simulink model "half_car_model_active_suspension_bump_brik"  (R2023b)
settings: Solver=VariableStepAuto  StartTime=0.0  StopTime=20  RelTol=1e-3
values from neighbouring files (symbols this model uses):
  e0 = [0; 0]    [half_car_active_suspensions_bump_brik.m]
  p = [ m ... (first row only)    [parameters.m]
  r0 = [Delta0 ... (first row only)    [half_car_active_suspensions_bump_brik.m]
  u0 = [0 ... (first row only)    [half_car_active_suspensions_bump_brik.m]    (also in prova_ordinata.m = [0; k * Delta0 * (df - dr)]; prova_ordinata_novembre.m = [0; k * Delta0 * (df - dr)])
  x0 = [Delta0 ... (first row only)    [half_car_active_suspensions_bump_brik.m]    (also in prova.m = [  -m*g/(2*k); prova_ordinata.m; prova_ordinata_novembre.m = [Delta0; 0; 0; 0; 0; 0; 0; 0])
  x0_lin = [ ... (first row only)    [half_car_active_suspensions_bump_brik.m]
  y0 = [0 ... (first row only)    [half_car_active_suspensions_bump_brik.m]
libraries: simulink x1
settings Model: Creator=alex2  LastModifiedBy=alex2

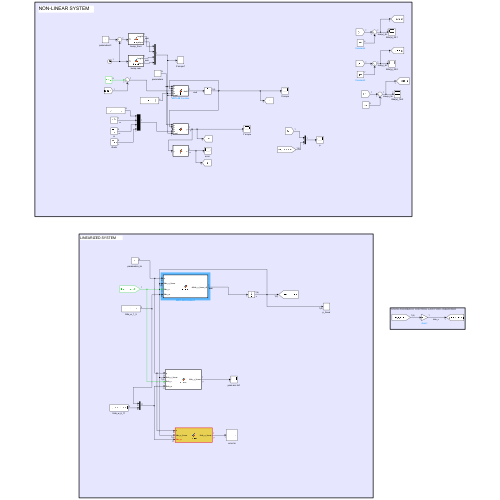
[thumbnail: Simulink's stored preview of the top-level diagram]
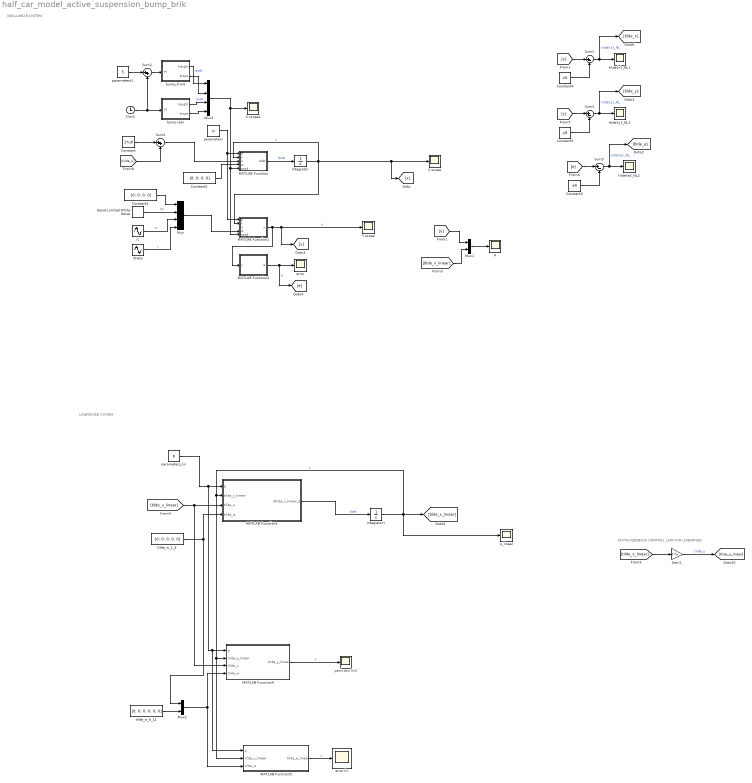
== system half_car_model_active_suspension_bump_brik ==
  note: LINEARIZED SYSTEM
  note: NON-LINEAR SYSTEM
  note: STATE-FEEDBACK CONTROL LAW FOR LINEARISED
  " error lin" : Scope
  Band-Limited White Noise : simulink/Sources/Band-Limited White Noise  Cov="1*[0.00001*1e-2; 0.00001*1e-2;  0.00001*1e-2; 0.00001*1e-2; 0.00001*1e-2]"  Ts=1e-2  seed=[23341; 31826; 11111; 81818; 00001]
  Clock : Clock
  Constant : Constant  Value=1*u0
  Constant1 : Constant  Value=[0; 0; 0; 0]
  Constant2 : Constant  Value=[0; 0; 0; 0]
  Constant3 : Constant  Value=y0
  Constant4 : Constant  Value=x0
  Constant5 : Constant  Value=e0
  Gain1 : Gain  Gain=0  Multiplication=Matrix(K*u)
  Integrator : Integrator  InitialCondition=x0
  Integrator1 : Integrator  InitialCondition=x0_lin
  MATLAB Function : MATLAB Function  TreatAsAtomicUnit=on
  MATLAB Function1 : MATLAB Function  TreatAsAtomicUnit=on
  MATLAB Function2 : MATLAB Function  TreatAsAtomicUnit=on
  MATLAB Function3 : MATLAB Function  TreatAsAtomicUnit=on
  MATLAB Function4 : MATLAB Function  TreatAsAtomicUnit=on
  MATLAB Function5 : MATLAB Function  TreatAsAtomicUnit=on
  Mux : Mux
  Mux1 : Mux  Inputs=2
  Mux2 : Mux  Inputs=2
  Mux3 : Mux
  Sum1 : Sum  Inputs=|+-
  Sum2 : Sum  Inputs=|++
  Sum3 : Sum  Inputs=|+-
  Sum4 : Sum  Inputs=|++
  Sum5 : Sum  Inputs=|+-
  X scope : Scope
  X scope1 : Scope
  Y scope : Scope
  bump rear : MATLAB Function  TreatAsAtomicUnit=on
  bump_front : MATLAB Function  TreatAsAtomicUnit=on
  "error " : Scope
  p : Scope
  p_linear : Scope
  parameters : Constant  Value=p
  parameters1 : Constant  Value=5
  parameters_lin : Constant  Value=p
  rtheta : Sin  Amplitude=0  Bias=r0  Frequency=0  SampleTime=0
  rz : Sin  Amplitude=0  Bias=r0  Frequency=0  SampleTime=0
  tilde_w_1_5 : Constant  Value=[0; 0; 0; 0; 0]
  tilde_w_6_11 : Constant  Value=[0; 0; 0; 0; 0; 0]
  "tilde{e}_NL2" : Scope
  "tilde{x}_NL1" : Scope
  "tilde{y}_NL2" : Scope
  yaxis acc lin1 : Scope
  wires:
  MATLAB Function/1(dxdt) -> Integrator/1  "dxdt"
  Integrator/1 -> MATLAB Function1/2(x), [x], X scope/1, MATLAB Function/2(x)  "x"
  Band-Limited White Noise/1 -> Mux/2  "nu"
  rz/1 -> Mux/3  "rz"
  Constant1/1 -> Mux/1
  Mux/1 -> MATLAB Function1/4(w)
  Constant2/1 -> MATLAB Function/4(w)
  MATLAB Function1/1(y) -> Y scope/1, [y], MATLAB Function2/1(y)  "y"
  rtheta/1 -> Mux/4  "r"
  MATLAB Function2/1(e) -> [e], "error "/1  "e"
  tilde_w_1_5/1 -> Mux2/1, MATLAB Function3/4(tilde_w)
  [tilde_u_linear] -> MATLAB Function4/3(tilde_u), MATLAB Function3/3(tilde_u)
  MATLAB Function3/1(dtilde_x_linear_dt) -> Integrator1/1  "dxdt"
  Integrator1/1 -> p_linear/1, MATLAB Function5/2(tilde_x_linear), MATLAB Function4/2(tilde_x_linear), MATLAB Function3/2(tilde_x_linear), [tilde_x_linear]  "x"
  parameters/1 -> MATLAB Function1/1(p), MATLAB Function/1(p)
  parameters_lin/1 -> MATLAB Function5/1(p), MATLAB Function4/1(p), MATLAB Function3/1(p)
  Mux2/1 -> MATLAB Function4/4(tilde_w), MATLAB Function5/3(tilde_w)
  tilde_w_6_11/1 -> Mux2/2
  MATLAB Function5/1(tilde_e_linear) -> " error lin"/1  "y"
  [tilde_u] -> Sum4/2
  Constant/1 -> Sum4/1
  Sum4/1 -> MATLAB Function/3(u)
  Sum1/1 -> [tilde_x], "tilde{x}_NL1"/1  "tilde{x}_NL"
  [x] -> Sum1/1
  Constant4/1 -> Sum1/2
  Gain1/1 -> [tilde_u_linear]  "tilde_u"
  [tilde_x_linear] -> Gain1/1
  MATLAB Function4/1(tilde_y_linear) -> yaxis acc lin1/1  "y"
  Mux1/1 -> p/1
  [x] -> Mux1/1
  [tilde_x_linear] -> Mux1/2
  Mux3/1 -> MATLAB Function/5(road), MATLAB Function1/5(road), X scope1/1
  Clock/1 -> Sum2/2, bump rear/1(Tf)
  bump rear/1(height) -> Mux3/3  "dxdt"
  bump rear/2(slope) -> Mux3/4
  bump_front/2(slope) -> Mux3/2
  bump_front/1(height) -> Mux3/1  "dxdt"
  Sum2/1 -> bump_front/1(Tf)
  parameters1/1 -> Sum2/1
  [y] -> Sum3/1
  Sum3/1 -> [tilde_y], "tilde{y}_NL2"/1  "tilde{y}_NL"
  Constant3/1 -> Sum3/2
  [e] -> Sum5/1
  Sum5/1 -> [tilde_e], "tilde{e}_NL2"/1  "tilde{e}_NL"
  Constant5/1 -> Sum5/2

== matlab function half_car_model_active_suspension_bump_brik/MATLAB Function1 ==
  data: p input; x input; u input; y output; w input; road input
function y = h(p,x, u, w, road)

%% parameters
m = p(1);      % [kg] mass
k = p(2);    % [N/m] spring stiffness
beta = p(3);   % [N/(m/s)] damper coeff.
ell0 = p(4);   % [m] 0-load lenght
g = p(5);   % [m/s^2] gravity acceleration
df = p(6);     % [m] distance between center of mass and front
dr = p(7);     % [m] distance between center of mass and rear
J = p(8);      % [kg*m^2] Moment of intertia

%% state
pz = x(1);        % [m] heigth of the center of mass of the car 
vz = x(2);        % [m/s] speed of the center of mass of the car 
ptheta = x(3);    % [Rad] pitch angle of the car 
vtheta = x(4);    % [Rad/s] angular speed of the car 
thetaroad_f = road(3); % [Rad]Road slope
zroad_f = road(4);     %[m]Road height 
thetaroad_r = -road(1); % [Rad]Road slope
zroad_r = road(2);     %[m]Road height 
%% state evolution

s1 = pz+df*(sin(ptheta)-sin(thetaroad_f)); % height of front suspension
s3 = pz-dr*(sin(ptheta)-sin(thetaroad_r)); % height of rear suspension

s2 = vz+df*(vtheta*cos(ptheta)-zroad_f*cos(thetaroad_f)); % height speed of front suspension
s4 = vz-dr*(vtheta*cos(ptheta)-zroad_r*cos(thetaroad_r)); % height speed of rear suspension


lf = s1 + ell0;
lr = s3 + ell0;

%f2 = -g + (((-k*(s1-ell0)-beta*s2)+(-k*(s3-ell0)-beta*s4))+u(1))/m; %  con ell0
%f4 = (df*(-k*(s1-ell0)-beta*s2)-dr*(-k*(s3-ell0)-beta*s4)+u(2)+fwfront*lf+fwrear*lr)/J; %

f2 = -g + (((-k*(s1)-beta*s2)+(-k*(s3)-beta*s4))+u(1))/m; % senza ell0
%f4 = (df*(-k*(s1)-beta*s2)-dr*(-k*(s3)-beta*s4)+u(2)+fwfront*lf+fwrear*lr)/J; %


zgsecond = w(1);
alphag = w(2);
fwfront = w(3);
fwrear = w(4);
nuy = w(5);
nuz = w(6);
nug = w(7);
nuf = w(8);
nur = w(9);

%% reference
rz = w(10);
rtheta=w(11);


%% output
y = [sin(x(3))*(f2 + g) + cos(x(3)) * ((fwrear + fwfront) / m)+nuy; 
     cos(x(3))*(f2 + g) - sin(x(3)) * ((fwrear + fwfront) / m)+nuz; %se facciamo cosi ci da in condizioni stazionarie Zaxisacc=9.81, se vogliamo il valore negativo mettere "-" davanti a coseno 
     x(4)+nug;
     s1+nuf;
     s3+nur;
     rz;
     rtheta];
end

== matlab function half_car_model_active_suspension_bump_brik/MATLAB Function ==
  data: p input; x input; u input; dxdt output; w input; road input
function dxdt = f(p,x,u,w,road)
%% parameters
%% parameters
m = p(1);      % [kg] mass
k = p(2);    % [N/m] spring stiffness
beta = p(3);   % [N/(m/s)] damper coeff.
ell0 = p(4);   % [m] 0-load lenght
g = p(5);   % [m/s^2] gravity acceleration
df = p(6);     % [m] distance between center of mass and front
dr = p(7);     % [m] distance between center of mass and rear
J = p(8);      % [kg*m^2] Moment of interti
%% state
pz = x(1);        % [m] heigth of the center of mass of the car 
vz = x(2);        % [m/s] speed of the center of mass of the car 
ptheta = x(3);    % [Rad] pitch angle of the car 
vtheta = x(4);    % [Rad/s] angular speed of the car 
thetaroad_f = road(3); % [Rad]Road slope
zroad_f = road(4);     %[m]Road height 

thetaroad_r = -road(1); % [Rad]Road slope
zroad_r = road(2);     %[m]Road height 

%% disturbance
zgsecond = w(1);
alphag = w(2);
fwfront = w(3);
fwrear = w(4);

%todo: Vedere se servono due disturbi 

%% state evolution
 
s1 = pz+df*(sin(ptheta)-sin(thetaroad_f)); % height of front suspension
s3 = pz-dr*(sin(ptheta)-sin(thetaroad_r)); % height of rear suspension

s2 = vz+df*(vtheta*cos(ptheta)-zroad_f*cos(thetaroad_f)); % height speed of front suspension
s4 = vz-dr*(vtheta*cos(ptheta)-zroad_r*cos(thetaroad_r)); % height speed of rear suspension

lf = s1 + ell0;
lr = s3 + ell0;

%f2 = -g + (((-k*(s1-ell0)-beta*s2)+(-k*(s3-ell0)-beta*s4))+u(1))/m; %  con  ell0
%f4 = (df*(-k*(s1-ell0)-beta*s2)-dr*(-k*(s3-ell0)-beta*s4)+u(2)+fwfront*lf+fwrear*lr)/J; %


f2 = -g + (((-k*(s1)-beta*s2)+(-k*(s3)-beta*s4))+u(1))/m; %  senza ell0
f4 = (df*(-k*(s1)-beta*s2)-dr*(-k*(s3)-beta*s4)+u(2)+fwfront*lf+fwrear*lr)/J; %

dxdt = [vz;
        f2-zgsecond; 
        x(4);
        f4;
        x(6);
        alphag];
        




end

== matlab function half_car_model_active_suspension_bump_brik/MATLAB Function2 ==
  data: y input; e output
function e = E(y)

df = 1;     % [m] distance between center of mass and front
dr = 1;     % [m] distance between center of mass and rear


yy = y(1); % output of h block yaxisacc 
yz = y(2); % output of h block zaxisacc 
yg = y(3); % output of h block gyro
yf = y(4); % output of h block pot. front
yr = y(5); % output of h block pot. rear
 
%% ref
rz = y(6);
rtheta = y(7);

e = [
    (yf*dr+yr*df)/(dr+df)-rz; 
    asin((yy)/(sqrt(yy^2+yz^2)))-rtheta];
end

== matlab function half_car_model_active_suspension_bump_brik/MATLAB Function3 ==
  data: p input; tilde_x_linear input; tilde_u input; dtilde_x_linear_dt output; tilde_w input

function dtilde_x_linear_dt = Linear(p,tilde_x_linear,tilde_u,tilde_w)





%% parameters
m = p(1);      % [kg] mass
k = p(2);    % [N/m] spring stiffness
beta = p(3);   % [N/(m/s)] damper coeff.
ell0 = p(4);   % [m] 0-load lenght
g = p(5);   % [m/s^2] gravity acceleration
df = p(6);     % [m] distance between center of mass and front
dr = p(7);     % [m] distance between center of mass and rear
J = p(8);      % [kg*m^2] Moment of interti


delta0 = -m*g/(2*k);
A = [ 0, 1, 0, 0, 0, 0;
      -(2*k)/m, -(2*beta)/m, -(df*k - dr*k)/m, -(beta*df - beta*dr)/m, 0 ,0;
      0, 0, 0, 1;
      -(df*k - dr*k)/J, -(beta*df - beta*dr)/J, -(k*df^2 + k*dr^2)/J, -(beta*df^2 + beta*dr^2)/J, 0 , 0;
      0, 0, 0, 0, 0, 0;
      0, 0, 0, 0, 0 ,0];

B1 = [ 0, 0;
       1/m, 0;
       0, 0;
       0, 1/J;
       0, 0;
       0, 0];

B2 = [ 0, 0, 0, 0;
       -1, 0, 0, 0;
       0, 0, 0, 0;
       0, 0, (ell0 - (g*m)/(2*k))/J, (ell0 - (g*m)/(2*k))/J;
       0, 0, 0, 0;
       0, 1, 0, 0];




%% state evolution
dtilde_x_linear_dt = A*tilde_x_linear+B1*tilde_u+B2*tilde_w;
end

== matlab function half_car_model_active_suspension_bump_brik/MATLAB Function4 ==
  data: p input; tilde_x_linear input; tilde_u input; tilde_y_linear output; tilde_w input
function tilde_y_linear = Linear(p,tilde_x_linear,tilde_u,tilde_w)


%% parameters
m = p(1);      % [kg] mass
k = p(2);    % [N/m] spring stiffness
beta = p(3);   % [N/(m/s)] damper coeff.
ell0 = p(4);   % [m] 0-load lenght
g = p(5);   % [m/s^2] gravity acceleration
df = p(6);     % [m] distance between center of mass and front
dr = p(7);     % [m] distance between center of mass and rear
J = p(8);      % [kg*m^2] Moment of interti



C = [0, 0, g, 0, 0, 0;
    -2*k/m, -2*beta/m, -k*(df-dr)/m, -beta*(df-dr)/m, k*(df-dr)/m, beta*(df-dr)/m;
    0, 0, 0, 1, 0, 0;
    1, 0, df, 0, -df, 0;
    1, 0, -dr, 0, dr, 0];


D1 = [0,0;
     1/m, 0;
     0,0;
     0,0;
     0,0];

D2 = [0,0,1/m,1/m,1,0,0,0,0,0,0;
      0,0,0,0,0,1,0,0,0,0,0;
      0,0,0,0,0,0,1,0,0,0,0;
      0,0,0,0,0,0,0,1,0,0,0;
      0,0,0,0,0,0,0,0,1,0,0];




%% state evolution
tilde_y_linear = C*tilde_x_linear+D1*tilde_u+D2*tilde_w;
end

== matlab function half_car_model_active_suspension_bump_brik/MATLAB Function5 ==
  data: p input; tilde_x_linear input; tilde_e_linear output; tilde_w input
function tilde_e_linear = Linear(p,tilde_x_linear,tilde_w)


%% parameters
m = p(1);      % [kg] mass
k = p(2);    % [N/m] spring stiffness
beta = p(3);   % [N/(m/s)] damper coeff.
ell0 = p(4);   % [m] 0-load lenght
g = p(5);   % [m/s^2] gravity acceleration
df = p(6);     % [m] distance between center of mass and front
dr = p(7);     % [m] distance between center of mass and rear
J = p(8);      % [kg*m^2] Moment of interti



Ce = [1,0,0,0,0,0;
      0,0,1,0,0,0];



De2 = [0,0,0,0,0,0,0,dr/(dr+df),df/(dr+df),-1,0;
       0,0, 1/(m*g),1/(m*g),1/g,0,0,0,0,0,-1];




%% state evolution
tilde_e_linear = Ce*tilde_x_linear+De2*tilde_w;
end

== matlab function half_car_model_active_suspension_bump_brik/bump rear ==
  data: height output; slope output; Tf input
function [height, slope] = bump(Tf)
    % Parametri
    a = 0.5;       % Ampiezza del bump (m)
    V = 20;         % Velocità del veicolo (m/s)
    lambda = 5;     % Lunghezza dell'onda del bump (m)
    Tspan = 5;      % Durata della simulazione (s)
    T1 = 5;         % Tempo di inizio del bump
    T2 = T1 + lambda/V; % Tempo di fine del bump

    % Calcola l'altezza della strada in base alla funzione del bump
    % Sostituzione di heaviside con un controllo manuale
    height = (a/2) * (1 - cos((2*pi*V*Tf)/lambda)) .* (Tf >= T1 & Tf <= T2); 
    
    % Calcola la pendenza della strada (derivata prima dell'altezza rispetto al tempo)
    slope = (a/2) * (2*pi*V/lambda) .* sin((2*pi*V*Tf)/lambda) .* (Tf >= T1 & Tf <= T2); 
end

== matlab function half_car_model_active_suspension_bump_brik/bump_front ==
  data: height output; slope output; Tf input
function [height, slope] = bump(Tf)
    % Parametri
    a = 0.5;       % Ampiezza del bump (m)
    V = 20;         % Velocità del veicolo (m/s)
    lambda = 5;     % Lunghezza dell'onda del bump (m)
    Tspan = 5;      % Durata della simulazione (s)
    T1 = 5;         % Tempo di inizio del bump
    T2 = T1 + lambda/V; % Tempo di fine del bump

    % Calcola l'altezza della strada in base alla funzione del bump
    % Sostituzione di heaviside con un controllo manuale
    height = (a/2) * (1 - cos((2*pi*V*Tf)/lambda)) .* (Tf >= T1 & Tf <= T2); 
    
    % Calcola la pendenza della strada (derivata prima dell'altezza rispetto al tempo)
    slope = (a/2) * (2*pi*V/lambda) .* sin((2*pi*V*Tf)/lambda) .* (Tf >= T1 & Tf <= T2); 
end
